simulink model "IIR_Transposed_Direct_Form_II"  (R2012b)
settings: Solver=ode45  StartTime=0.0  StopTime=10.0  RelTol=1e-3
settings Model: Creator=Ahmad  LastModifiedBy=Ahmad

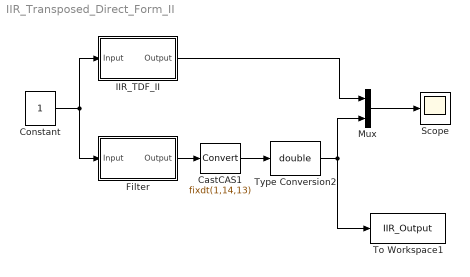
== system IIR_Transposed_Direct_Form_II ==
  CastCAS1 : DataTypeConversion  OutDataTypeStr=fixdt(1,14,13)  SaturateOnIntegerOverflow=on
  Constant : Constant  VectorParams1D=off  OutDataTypeStr=double  SampleTime=1/50e6
  Filter : Subsystem  Tag=FilterWizardSubSystem
      settings: ErrorFcn=dspFilterRealizedInBasicElemsAlgLoopErrFcnCallback
  IIR_TDF_II : Subsystem  Tag=FilterWizardSubSystem
      settings: ErrorFcn=dspFilterRealizedInBasicElemsAlgLoopErrFcnCallback
  Mux : Mux  Inputs=2
  Scope : Scope
      settings: YMin=0.1  YMax=0.85
  To Workspace1 : ToWorkspace  VariableName=IIR_Output  SampleTime=-1  SaveFormat=Timeseries
  Type Conversion2 : DataTypeConversion  OutDataTypeStr=double
  wires:
  Constant/1 -> Filter/1(Input), IIR_TDF_II/1(Input)
  Filter/1(Output) -> CastCAS1/1
  Mux/1 -> Scope/1
  IIR_TDF_II/1(Output) -> Mux/1
  Type Conversion2/1 -> To Workspace1/1, Mux/2
  CastCAS1/1 -> Type Conversion2/1

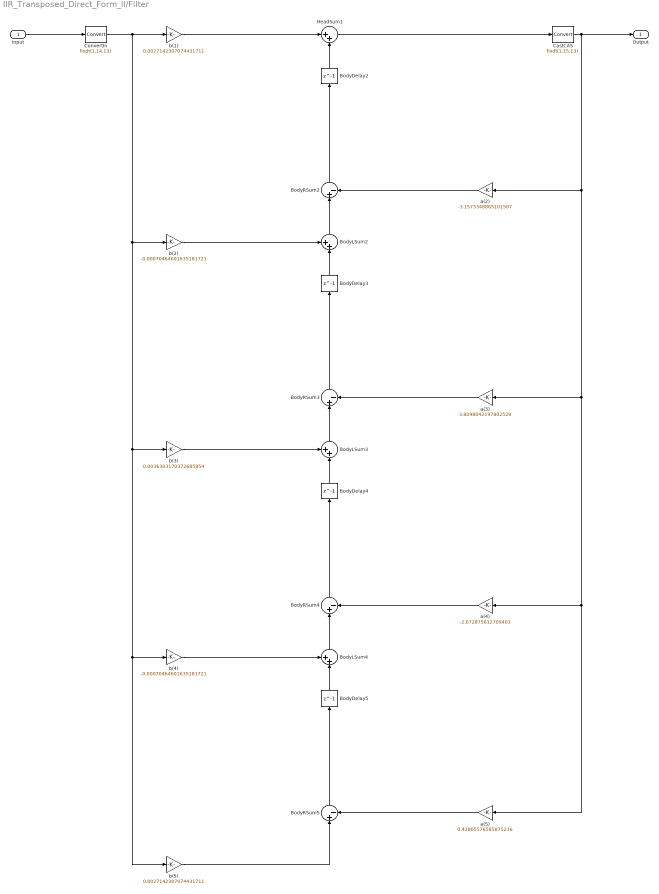
== system IIR_Transposed_Direct_Form_II/Filter ==
  Input : Inport
  BodyDelay{2..5} (4 alike) : Delay  DelayLength=1  InitialCondition=0
  BodyLSum2 : Sum  Inputs=++|  AccumDataTypeStr=fixdt(1,31,27)  OutDataTypeStr=fixdt(1,31,27)
  BodyLSum3 : Sum  Inputs=++|  AccumDataTypeStr=fixdt(1,31,27)  OutDataTypeStr=fixdt(1,31,27)
  BodyLSum4 : Sum  Inputs=++|  AccumDataTypeStr=fixdt(1,31,27)  OutDataTypeStr=fixdt(1,31,27)
  BodyRSum{2..5} (4 alike) : Sum  Inputs=|+-  AccumDataTypeStr=fixdt(1,31,27)  OutDataTypeStr=fixdt(1,31,27)
  CastCAS : DataTypeConversion  OutDataTypeStr=fixdt(1,15,13)
  ConvertIn : DataTypeConversion  OutDataTypeStr=fixdt(1,14,13)  RndMeth=Nearest  SaturateOnIntegerOverflow=on
  HeadSum1 : Sum  Inputs=|++  AccumDataTypeStr=fixdt(1,31,27)  OutDataTypeStr=fixdt(1,31,27)
  a(2) : Gain  Gain=-3.1573348865101507  ParamDataTypeStr=fixdt(1,17,14)  OutDataTypeStr=fixdt(1,31,27)
  a(3) : Gain  Gain=3.8098042197802529  ParamDataTypeStr=fixdt(1,17,14)  OutDataTypeStr=fixdt(1,31,27)
  a(4) : Gain  Gain=-2.072875612709403  ParamDataTypeStr=fixdt(1,17,14)  OutDataTypeStr=fixdt(1,31,27)
  a(5) : Gain  Gain=0.42805576585875216  ParamDataTypeStr=fixdt(1,17,14)  OutDataTypeStr=fixdt(1,31,27)
  b(1) : Gain  Gain=0.0027142307074431711  ParamDataTypeStr=fixdt(1,17,14)  OutDataTypeStr=fixdt(1,31,27)
  b(2) : Gain  Gain=-0.00070464601635181721  ParamDataTypeStr=fixdt(1,17,14)  OutDataTypeStr=fixdt(1,31,27)
  b(3) : Gain  Gain=0.0036303170372685854  ParamDataTypeStr=fixdt(1,17,14)  OutDataTypeStr=fixdt(1,31,27)
  b(4) : Gain  Gain=-0.00070464601635181721  ParamDataTypeStr=fixdt(1,17,14)  OutDataTypeStr=fixdt(1,31,27)
  b(5) : Gain  Gain=0.0027142307074431711  ParamDataTypeStr=fixdt(1,17,14)  OutDataTypeStr=fixdt(1,31,27)
  Output : Outport
  wires:
  Input/1 -> ConvertIn/1
  b(1)/1 -> HeadSum1/1
  HeadSum1/1 -> CastCAS/1
  CastCAS/1 -> a(4)/1, a(5)/1, a(3)/1, a(2)/1, Output/1
  ConvertIn/1 -> b(4)/1, b(5)/1, b(3)/1, b(2)/1, b(1)/1
  b(2)/1 -> BodyLSum2/1
  BodyLSum2/1 -> BodyRSum2/1
  BodyRSum2/1 -> BodyDelay2/1
  a(2)/1 -> BodyRSum2/2
  BodyDelay2/1 -> HeadSum1/2
  b(3)/1 -> BodyLSum3/1
  BodyLSum3/1 -> BodyRSum3/1
  BodyRSum3/1 -> BodyDelay3/1
  a(3)/1 -> BodyRSum3/2
  BodyDelay3/1 -> BodyLSum2/2
  b(4)/1 -> BodyLSum4/1
  BodyLSum4/1 -> BodyRSum4/1
  BodyRSum4/1 -> BodyDelay4/1
  a(4)/1 -> BodyRSum4/2
  BodyDelay4/1 -> BodyLSum3/2
  b(5)/1 -> BodyRSum5/1
  BodyRSum5/1 -> BodyDelay5/1
  a(5)/1 -> BodyRSum5/2
  BodyDelay5/1 -> BodyLSum4/2

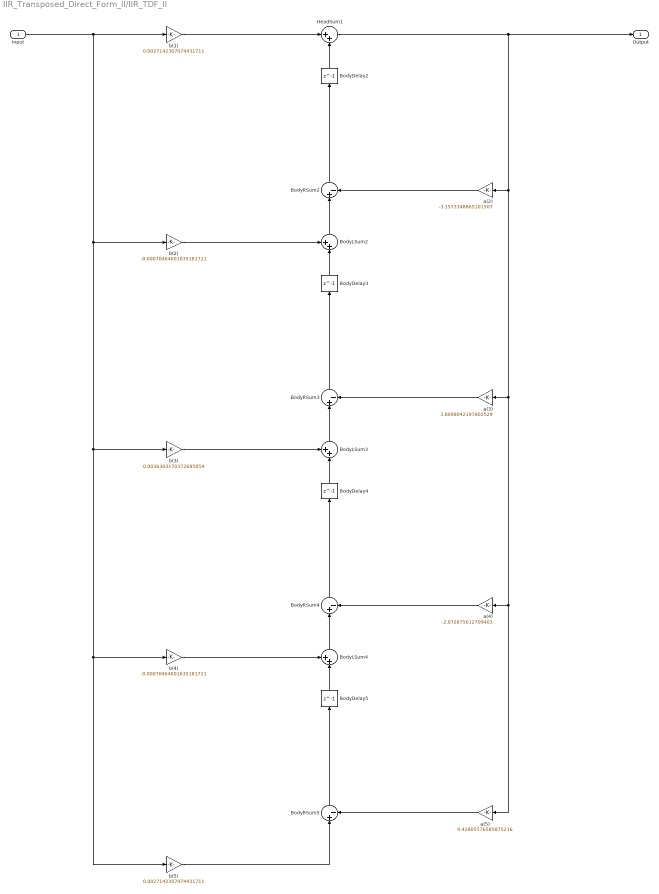
== system IIR_Transposed_Direct_Form_II/IIR_TDF_II ==
  Input : Inport
  BodyDelay{2..5} (4 alike) : Delay  DelayLength=1  InitialCondition=0
  BodyLSum2 : Sum  Inputs=++|  RndMeth=Nearest  SaturateOnIntegerOverflow=on  OutDataTypeStr=Inherit: Same as first input
  BodyLSum3 : Sum  Inputs=++|  RndMeth=Nearest  SaturateOnIntegerOverflow=on  OutDataTypeStr=Inherit: Same as first input
  BodyLSum4 : Sum  Inputs=++|  RndMeth=Nearest  SaturateOnIntegerOverflow=on  OutDataTypeStr=Inherit: Same as first input
  BodyRSum{2..5} (4 alike) : Sum  Inputs=|+-  RndMeth=Nearest  SaturateOnIntegerOverflow=on  OutDataTypeStr=Inherit: Same as first input
  HeadSum1 : Sum  Inputs=|++  RndMeth=Nearest  SaturateOnIntegerOverflow=on  OutDataTypeStr=Inherit: Same as first input
  a(2) : Gain  Gain=-3.1573348865101507  ParamDataTypeStr=double  RndMeth=Nearest  SaturateOnIntegerOverflow=on  OutDataTypeStr=Inherit: Same as input
  a(3) : Gain  Gain=3.8098042197802529  ParamDataTypeStr=double  RndMeth=Nearest  SaturateOnIntegerOverflow=on  OutDataTypeStr=Inherit: Same as input
  a(4) : Gain  Gain=-2.072875612709403  ParamDataTypeStr=double  RndMeth=Nearest  SaturateOnIntegerOverflow=on  OutDataTypeStr=Inherit: Same as input
  a(5) : Gain  Gain=0.42805576585875216  ParamDataTypeStr=double  RndMeth=Nearest  SaturateOnIntegerOverflow=on  OutDataTypeStr=Inherit: Same as input
  b(1) : Gain  Gain=0.0027142307074431711  ParamDataTypeStr=double  RndMeth=Nearest  SaturateOnIntegerOverflow=on  OutDataTypeStr=Inherit: Same as input
  b(2) : Gain  Gain=-0.00070464601635181721  ParamDataTypeStr=double  RndMeth=Nearest  SaturateOnIntegerOverflow=on  OutDataTypeStr=Inherit: Same as input
  b(3) : Gain  Gain=0.0036303170372685854  ParamDataTypeStr=double  RndMeth=Nearest  SaturateOnIntegerOverflow=on  OutDataTypeStr=Inherit: Same as input
  b(4) : Gain  Gain=-0.00070464601635181721  ParamDataTypeStr=double  RndMeth=Nearest  SaturateOnIntegerOverflow=on  OutDataTypeStr=Inherit: Same as input
  b(5) : Gain  Gain=0.0027142307074431711  ParamDataTypeStr=double  RndMeth=Nearest  SaturateOnIntegerOverflow=on  OutDataTypeStr=Inherit: Same as input
  Output : Outport
  wires:
  Input/1 -> b(4)/1, b(5)/1, b(3)/1, b(2)/1, b(1)/1
  b(1)/1 -> HeadSum1/1
  HeadSum1/1 -> a(4)/1, a(5)/1, a(3)/1, a(2)/1, Output/1
  b(2)/1 -> BodyLSum2/1
  BodyLSum2/1 -> BodyRSum2/1
  BodyRSum2/1 -> BodyDelay2/1
  a(2)/1 -> BodyRSum2/2
  BodyDelay2/1 -> HeadSum1/2
  b(3)/1 -> BodyLSum3/1
  BodyLSum3/1 -> BodyRSum3/1
  BodyRSum3/1 -> BodyDelay3/1
  a(3)/1 -> BodyRSum3/2
  BodyDelay3/1 -> BodyLSum2/2
  b(4)/1 -> BodyLSum4/1
  BodyLSum4/1 -> BodyRSum4/1
  BodyRSum4/1 -> BodyDelay4/1
  a(4)/1 -> BodyRSum4/2
  BodyDelay4/1 -> BodyLSum3/2
  b(5)/1 -> BodyRSum5/1
  BodyRSum5/1 -> BodyDelay5/1
  a(5)/1 -> BodyRSum5/2
  BodyDelay5/1 -> BodyLSum4/2
